simulink library "typhoonPatterns"  (R2017b)
settings: Solver=VariableStepAuto  StartTime=0.0  StopTime=10.0  RelTol=1e-3
undefined symbols (not defined in the file or in its folder): c_clamp, C_l, c_picoup_seq, crun_sp_ind, cst_sp_ind, f, f_picoup, f_sp_ind, fc, Jm, L, L1, L2, L_l, l_picoup_seq, La_DC, Ld, Lf_DC, Llr1_ind, Llr2_ind, Llr_ind, llrm_sp_ind, Lls_ind, llsa_sp_ind, llsm_sp_ind, Lm, Lq, n1, n2, nanm_sp_ind, pms, R, R1, R2, r_clamp, R_l, r_picoup_seq, Ra_DC, Rf_DC, Rm, Rr1_ind, Rr2_ind, Rr_ind, rrm_sp_ind, rrun_sp_ind, Rs, Rs_ind, rsa_sp_ind, rsm_sp_ind, rst_sp_ind
libraries: powerlib x282
(part 2 of 3)

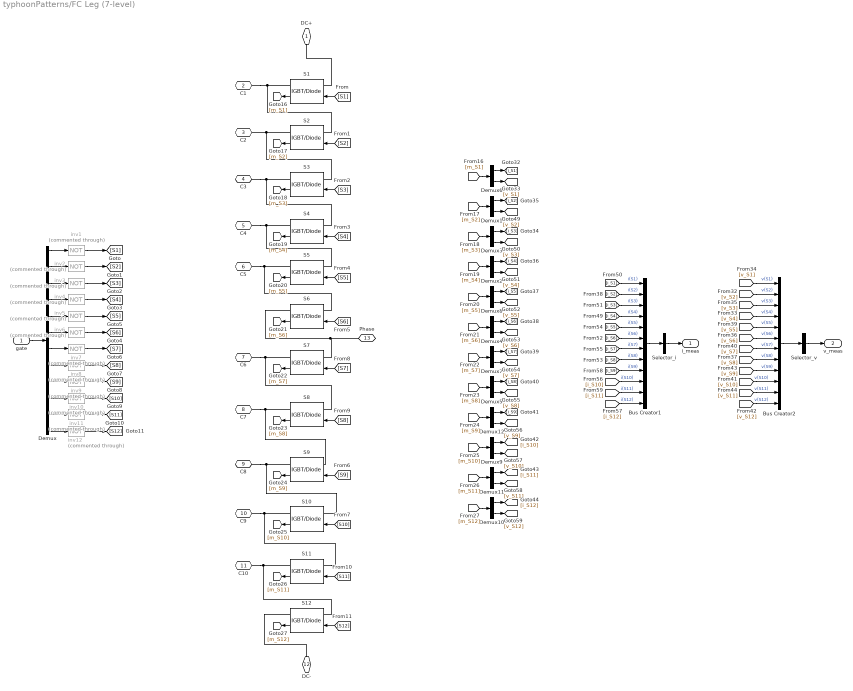
== system typhoonPatterns/FC Leg (7-level) ==
  gate : Inport
  Bus Creator1 : BusCreator  Inputs=12
  Bus Creator2 : BusCreator  Inputs=12
  Demux : Demux  Outputs=12
  Demux{1..12} (12 alike) : Demux  Outputs=2
  S{1..12} (12 alike) : powerlib/Power Electronics/IGBT//Diode  Ron=r_on  Rs=r_s  Cs=c_s  Measurements=on
  Selector_i : BusSelector  OutputSignals=i(S1)  OutputAsBus=on
  Selector_v : BusSelector  OutputSignals=v(S1)  OutputAsBus=on
  inv{1..12} (12 alike) : Logic  Commented=through  Operator=NOT  AllPortsSameDT=off  OutDataTypeStr=boolean
  DC+ : PMIOPort  Port=1  Side=Left
  C1 : PMIOPort  Port=2  Side=Left
  C2 : PMIOPort  Port=3  Side=Left
  C3 : PMIOPort  Port=4  Side=Left
  C4 : PMIOPort  Port=5  Side=Left
  C5 : PMIOPort  Port=6  Side=Left
  C6 : PMIOPort  Port=7  Side=Left
  C7 : PMIOPort  Port=8  Side=Left
  C8 : PMIOPort  Port=9  Side=Left
  C9 : PMIOPort  Port=10  Side=Left
  C10 : PMIOPort  Port=11  Side=Left
  DC- : PMIOPort  Port=12  Side=Left
  Phase : PMIOPort  Port=13  Side=Right
  i_meas : Outport
  v_meas : Outport  Port=2
  wires:
  Demux3/2 -> [v_S3]
  Demux1/1 -> [i_S2]
  [v_S7] -> Bus Creator2/7  "v(S7)"
  [v_S6] -> Bus Creator2/6  "v(S6)"
  Demux6/2 -> [v_S1]
  Demux6/1 -> [i_S1]
  [v_S1] -> Bus Creator2/1  "v(S1)"
  Bus Creator2/1 -> Selector_v/1
  Selector_v/1 -> v_meas/1
  Bus Creator1/1 -> Selector_i/1
  [v_S3] -> Bus Creator2/3  "v(S3)"
  [i_S2] -> Bus Creator1/2  "i(S2)"
  [i_S11] -> Bus Creator1/11  "i(S11)"
  [i_S4] -> Bus Creator1/4  "i(S4)"
  [i_S10] -> Bus Creator1/10  "i(S10)"
  [i_S1] -> Bus Creator1/1  "i(S1)"
  [i_S7] -> Bus Creator1/7  "i(S7)"
  [i_S5] -> Bus Creator1/5  "i(S5)"
  [i_S3] -> Bus Creator1/3  "i(S3)"
  [i_S12] -> Bus Creator1/12  "i(S12)"
  Demux7/1 -> [i_S7]
  Demux9/1 -> [i_S10]
  [m_S3] -> Demux3/1
  [v_S4] -> Bus Creator2/4  "v(S4)"
  Demux4/1 -> [i_S6]
  [m_S5] -> Demux8/1
  S2/1 -> [m_S2]
  [m_S11] -> Demux11/1
  [v_S8] -> Bus Creator2/8  "v(S8)"
  S12/1 -> [m_S12]
  S1/1 -> [m_S1]
  Demux5/1 -> [i_S8]
  Demux4/2 -> [v_S6]
  Demux2/2 -> [v_S4]
  inv7/1 -> [S7]
  inv8/1 -> [S8]
  inv6/1 -> [S6]
  inv12/1 -> [S12]
  Demux8/1 -> [i_S5]
  inv10/1 -> [S10]
  inv11/1 -> [S11]
  Demux11/1 -> [i_S11]
  Demux/1 -> inv1/1
  Demux/3 -> inv3/1
  [S5] -> S5/1
  [S6] -> S6/1
  S8/1 -> [m_S8]
  gate/1 -> Demux/1
  [S7] -> S7/1
  [i_S8] -> Bus Creator1/8  "i(S8)"
  Demux/4 -> inv4/1
  [S2] -> S2/1
  [i_S6] -> Bus Creator1/6  "i(S6)"
  Selector_i/1 -> i_meas/1
  [v_S5] -> Bus Creator2/5  "v(S5)"
  Demux/5 -> inv5/1
  [S11] -> S11/1
  [S4] -> S4/1
  Demux/12 -> inv12/1
  Demux/10 -> inv10/1
  [S9] -> S9/1
  Demux/8 -> inv8/1
  Demux/11 -> inv11/1
  Demux/9 -> inv9/1
  [i_S9] -> Bus Creator1/9  "i(S9)"
  [m_S9] -> Demux12/1
  [m_S6] -> Demux4/1
  S4/1 -> [m_S4]
  Demux1/2 -> [v_S2]
  S11/1 -> [m_S11]
  Demux/7 -> inv7/1
  [m_S8] -> Demux5/1
  Demux10/1 -> [i_S12]
  [m_S1] -> Demux6/1
  S5/1 -> [m_S5]
  [v_S10] -> Bus Creator2/10  "v(S10)"
  [v_S11] -> Bus Creator2/11  "v(S11)"
  [m_S7] -> Demux7/1
  Demux/6 -> inv6/1
  [v_S12] -> Bus Creator2/12  "v(S12)"
  S7/1 -> [m_S7]
  [m_S4] -> Demux2/1
  Demux12/2 -> [v_S9]
  inv5/1 -> [S5]
  S6/1 -> [m_S6]
  [m_S2] -> Demux1/1
  [S8] -> S8/1
  [S1] -> S1/1
  Demux3/1 -> [i_S3]
  Demux/2 -> inv2/1
  inv2/1 -> [S2]
  inv3/1 -> [S3]
  Demux5/2 -> [v_S8]
  Demux12/1 -> [i_S9]
  [v_S2] -> Bus Creator2/2  "v(S2)"
  [S10] -> S10/1
  inv1/1 -> [S1]
  S3/1 -> [m_S3]
  inv4/1 -> [S4]
  [m_S10] -> Demux9/1
  Demux10/2 -> [v_S12]
  Demux11/2 -> [v_S11]
  Demux2/1 -> [i_S4]
  [S12] -> S12/1
  Demux9/2 -> [v_S10]
  [m_S12] -> Demux10/1
  [v_S9] -> Bus Creator2/9  "v(S9)"
  Demux8/2 -> [v_S5]
  S10/1 -> [m_S10]
  Demux7/2 -> [v_S7]
  S9/1 -> [m_S9]
  [S3] -> S3/1
  inv9/1 -> [S9]
  connections:
  S7/LConn1 -- Phase/RConn1 -- S6/RConn1
  S8/LConn1 -- C6/RConn1 -- S7/RConn1
  C3/RConn1 -- S3/RConn1 -- S4/LConn1
  S8/RConn1 -- C7/RConn1 -- S9/LConn1
  C1/RConn1 -- S1/RConn1 -- S2/LConn1
  S6/LConn1 -- S5/RConn1 -- C5/RConn1
  C10/RConn1 -- S11/RConn1 -- S12/LConn1
  C2/RConn1 -- S2/RConn1 -- S3/LConn1
  S5/LConn1 -- S4/RConn1 -- C4/RConn1
  S10/LConn1 -- S9/RConn1 -- C8/RConn1
  C9/RConn1 -- S10/RConn1 -- S11/LConn1
  S1/LConn1 -- DC+/RConn1
  DC-/RConn1 -- S12/RConn1

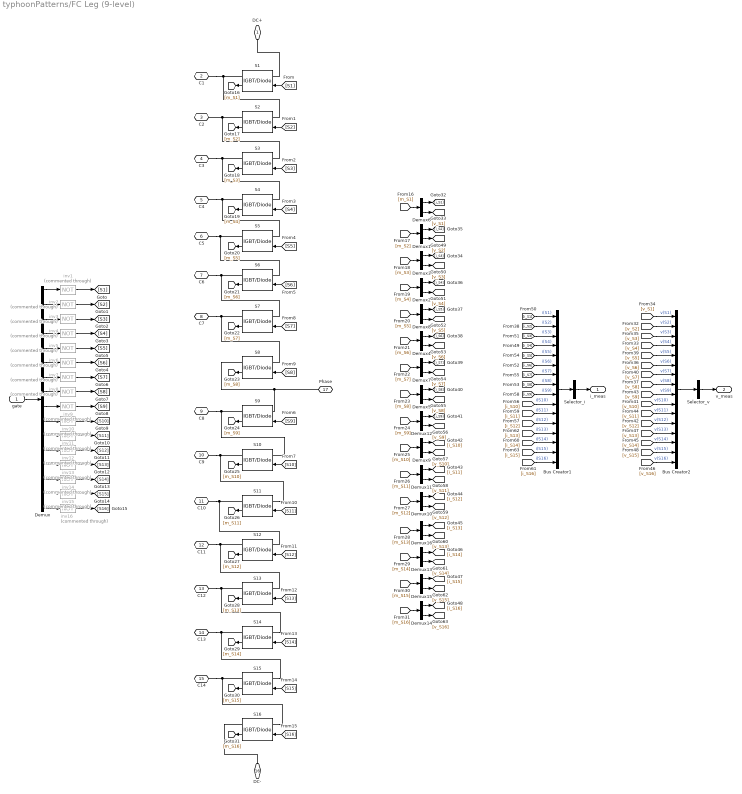
== system typhoonPatterns/FC Leg (9-level) ==
  gate : Inport
  Bus Creator1 : BusCreator  Inputs=16
  Bus Creator2 : BusCreator  Inputs=16
  Demux : Demux  Outputs=16
  Demux{1..16} (16 alike) : Demux  Outputs=2
  S{1..16} (16 alike) : powerlib/Power Electronics/IGBT//Diode  Ron=r_on  Rs=r_s  Cs=c_s  Measurements=on
  Selector_i : BusSelector  OutputSignals=i(S1)  OutputAsBus=on
  Selector_v : BusSelector  OutputSignals=v(S1)  OutputAsBus=on
  inv{1..16} (16 alike) : Logic  Commented=through  Operator=NOT  AllPortsSameDT=off  OutDataTypeStr=boolean
  DC+ : PMIOPort  Port=1  Side=Left
  C1 : PMIOPort  Port=2  Side=Left
  C2 : PMIOPort  Port=3  Side=Left
  C3 : PMIOPort  Port=4  Side=Left
  C4 : PMIOPort  Port=5  Side=Left
  C5 : PMIOPort  Port=6  Side=Left
  C6 : PMIOPort  Port=7  Side=Left
  C7 : PMIOPort  Port=8  Side=Left
  C8 : PMIOPort  Port=9  Side=Left
  C9 : PMIOPort  Port=10  Side=Left
  C10 : PMIOPort  Port=11  Side=Left
  C11 : PMIOPort  Port=12  Side=Left
  C12 : PMIOPort  Port=13  Side=Left
  C13 : PMIOPort  Port=14  Side=Left
  C14 : PMIOPort  Port=15  Side=Left
  DC- : PMIOPort  Port=16  Side=Left
  Phase : PMIOPort  Port=17  Side=Right
  i_meas : Outport
  v_meas : Outport  Port=2
  wires:
  Demux/15 -> inv15/1
  [S14] -> S14/1
  [S13] -> S13/1
  [S16] -> S16/1
  [S15] -> S15/1
  Demux/16 -> inv16/1
  Demux/14 -> inv14/1
  Demux/13 -> inv13/1
  Demux/12 -> inv12/1
  Demux/9 -> inv9/1
  Demux/2 -> inv2/1
  gate/1 -> Demux/1
  Demux/10 -> inv10/1
  [S11] -> S11/1
  [S12] -> S12/1
  Demux/8 -> inv8/1
  [S7] -> S7/1
  Demux/11 -> inv11/1
  [S8] -> S8/1
  [S5] -> S5/1
  [S3] -> S3/1
  Demux/4 -> inv4/1
  Demux/3 -> inv3/1
  [S9] -> S9/1
  Demux/7 -> inv7/1
  Demux/6 -> inv6/1
  Demux/1 -> inv1/1
  Demux/5 -> inv5/1
  [S4] -> S4/1
  [S6] -> S6/1
  [S2] -> S2/1
  [S1] -> S1/1
  [S10] -> S10/1
  inv1/1 -> [S1]
  inv3/1 -> [S3]
  inv4/1 -> [S4]
  inv2/1 -> [S2]
  inv5/1 -> [S5]
  inv8/1 -> [S8]
  inv6/1 -> [S6]
  inv7/1 -> [S7]
  inv9/1 -> [S9]
  inv11/1 -> [S11]
  inv10/1 -> [S10]
  inv12/1 -> [S12]
  inv15/1 -> [S15]
  inv13/1 -> [S13]
  inv14/1 -> [S14]
  inv16/1 -> [S16]
  S1/1 -> [m_S1]
  S2/1 -> [m_S2]
  S4/1 -> [m_S4]
  S5/1 -> [m_S5]
  S6/1 -> [m_S6]
  S3/1 -> [m_S3]
  S7/1 -> [m_S7]
  S8/1 -> [m_S8]
  S9/1 -> [m_S9]
  S10/1 -> [m_S10]
  S11/1 -> [m_S11]
  S12/1 -> [m_S12]
  S13/1 -> [m_S13]
  S14/1 -> [m_S14]
  S15/1 -> [m_S15]
  S16/1 -> [m_S16]
  [m_S1] -> Demux6/1
  Selector_v/1 -> v_meas/1
  Demux6/1 -> [i_S1]
  Bus Creator2/1 -> Selector_v/1
  [v_S1] -> Bus Creator2/1  "v(S1)"
  Selector_i/1 -> i_meas/1
  Demux6/2 -> [v_S1]
  [v_S2] -> Bus Creator2/2  "v(S2)"
  [v_S3] -> Bus Creator2/3  "v(S3)"
  [v_S4] -> Bus Creator2/4  "v(S4)"
  [v_S5] -> Bus Creator2/5  "v(S5)"
  [v_S7] -> Bus Creator2/7  "v(S7)"
  [v_S6] -> Bus Creator2/6  "v(S6)"
  [v_S8] -> Bus Creator2/8  "v(S8)"
  [v_S9] -> Bus Creator2/9  "v(S9)"
  [v_S11] -> Bus Creator2/11  "v(S11)"
  [v_S10] -> Bus Creator2/10  "v(S10)"
  [v_S12] -> Bus Creator2/12  "v(S12)"
  [v_S13] -> Bus Creator2/13  "v(S13)"
  [v_S15] -> Bus Creator2/15  "v(S15)"
  [v_S14] -> Bus Creator2/14  "v(S14)"
  [v_S16] -> Bus Creator2/16  "v(S16)"
  [i_S6] -> Bus Creator1/6  "i(S6)"
  [i_S5] -> Bus Creator1/5  "i(S5)"
  [i_S14] -> Bus Creator1/14  "i(S14)"
  [i_S7] -> Bus Creator1/7  "i(S7)"
  [i_S16] -> Bus Creator1/16  "i(S16)"
  [i_S13] -> Bus Creator1/13  "i(S13)"
  [i_S15] -> Bus Creator1/15  "i(S15)"
  [i_S1] -> Bus Creator1/1  "i(S1)"
  [i_S10] -> Bus Creator1/10  "i(S10)"
  [i_S8] -> Bus Creator1/8  "i(S8)"
  [i_S4] -> Bus Creator1/4  "i(S4)"
  [i_S11] -> Bus Creator1/11  "i(S11)"
  [i_S2] -> Bus Creator1/2  "i(S2)"
  [i_S12] -> Bus Creator1/12  "i(S12)"
  [i_S3] -> Bus Creator1/3  "i(S3)"
  [i_S9] -> Bus Creator1/9  "i(S9)"
  Bus Creator1/1 -> Selector_i/1
  Demux1/2 -> [v_S2]
  Demux1/1 -> [i_S2]
  [m_S2] -> Demux1/1
  Demux3/2 -> [v_S3]
  [m_S3] -> Demux3/1
  Demux2/1 -> [i_S4]
  Demux2/2 -> [v_S4]
  [m_S4] -> Demux2/1
  Demux8/2 -> [v_S5]
  Demux8/1 -> [i_S5]
  [m_S5] -> Demux8/1
  Demux4/1 -> [i_S6]
  Demux5/1 -> [i_S8]
  [m_S8] -> Demux5/1
  Demux4/2 -> [v_S6]
  [m_S6] -> Demux4/1
  Demux5/2 -> [v_S8]
  [m_S7] -> Demux7/1
  Demux7/2 -> [v_S7]
  Demux12/2 -> [v_S9]
  Demux12/1 -> [i_S9]
  [m_S9] -> Demux12/1
  Demux9/1 -> [i_S10]
  Demux10/1 -> [i_S12]
  [m_S12] -> Demux10/1
  Demux9/2 -> [v_S10]
  [m_S10] -> Demux9/1
  Demux10/2 -> [v_S12]
  [m_S11] -> Demux11/1
  Demux11/2 -> [v_S11]
  Demux16/2 -> [v_S13]
  Demux16/1 -> [i_S13]
  [m_S13] -> Demux16/1
  Demux13/1 -> [i_S14]
  Demux14/1 -> [i_S16]
  [m_S16] -> Demux14/1
  Demux13/2 -> [v_S14]
  [m_S14] -> Demux13/1
  Demux14/2 -> [v_S16]
  [m_S15] -> Demux15/1
  Demux15/2 -> [v_S15]
  Demux3/1 -> [i_S3]
  Demux7/1 -> [i_S7]
  Demux11/1 -> [i_S11]
  Demux15/1 -> [i_S15]
  connections:
  DC-/RConn1 -- S16/RConn1
  S1/LConn1 -- DC+/RConn1
  C1/RConn1 -- S1/RConn1 -- S2/LConn1
  S2/RConn1 -- S3/LConn1 -- C2/RConn1
  S8/RConn1 -- Phase/RConn1 -- S9/LConn1
  C3/RConn1 -- S3/RConn1 -- S4/LConn1
  S5/LConn1 -- S4/RConn1 -- C4/RConn1
  S6/LConn1 -- S5/RConn1 -- C5/RConn1
  C6/RConn1 -- S6/RConn1 -- S7/LConn1
  C7/RConn1 -- S7/RConn1 -- S8/LConn1
  S9/RConn1 -- C8/RConn1 -- S10/LConn1
  C9/RConn1 -- S10/RConn1 -- S11/LConn1
  C10/RConn1 -- S11/RConn1 -- S12/LConn1
  S13/LConn1 -- S12/RConn1 -- C11/RConn1
  S14/LConn1 -- S13/RConn1 -- C12/RConn1
  S15/LConn1 -- S14/RConn1 -- C13/RConn1
  S16/LConn1 -- S15/RConn1 -- C14/RConn1

== system typhoonPatterns/Flyback ==
  gate : Inport
  D : powerlib/Power Electronics/Diode  Ron=r_on  Lon=0  Vf=0  IC=0  UseSnubber=0  Rs=r_s  Cs=c_s  Measurements=off
  S : powerlib/Power Electronics/Mosfet  Ron=r_on  Lon=0  Rd=r_on  Vfd=0  IC=0  Rs=r_s  Cs=c_s  Measurements=off
  T : powerlib/Elements/Linear Transformer  UNITS=SI  NominalPower=[250e6 60 ]  winding1=[n1 R1 L1]  winding2=[n2 R2 L2]  ThreeWindings=off  winding3=[3.15e+05 0.7938 0.084225]  RmLm=[Rm Lm]  Measurements=None  DataType=on
  inv1 : Logic  Commented=through  Operator=NOT  AllPortsSameDT=off  OutDataTypeStr=boolean
  In+ : PMIOPort  Port=1  Side=Left
  In- : PMIOPort  Port=2  Side=Left
  Out+ : PMIOPort  Port=3  Side=Right
  Out- : PMIOPort  Port=4  Side=Right
  wires:
  inv1/1 -> S/1
  gate/1 -> inv1/1
  connections:
  In-/RConn1 -- S/RConn1
  S/LConn1 -- T/LConn2
  In+/RConn1 -- T/LConn1
  D/RConn1 -- Out+/RConn1
  D/LConn1 -- T/RConn2
  T/RConn1 -- Out-/RConn1

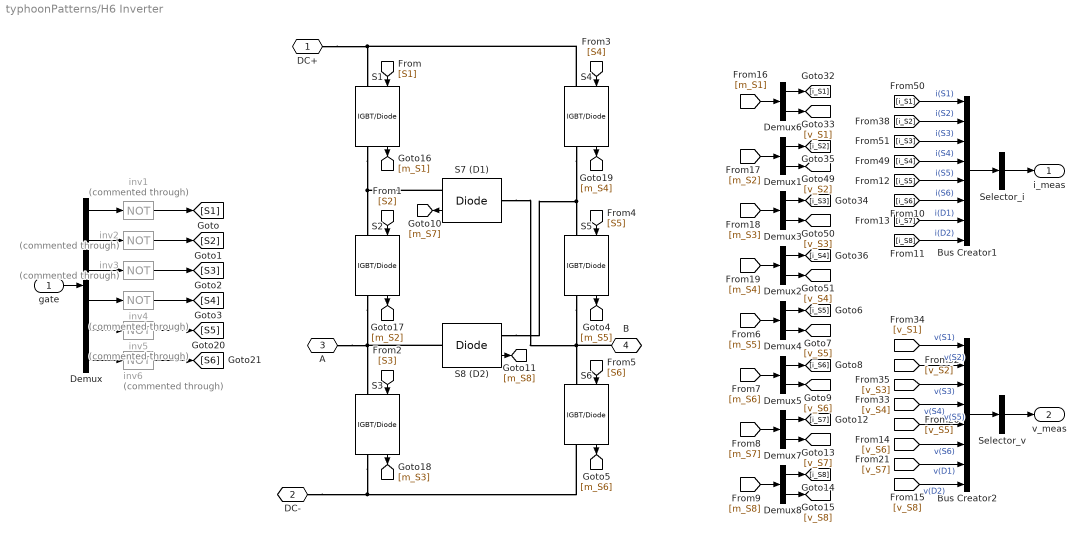
== system typhoonPatterns/H6 Inverter ==
  gate : Inport
  Bus Creator1 : BusCreator  Inputs=8
  Bus Creator2 : BusCreator  Inputs=8
  Demux : Demux  Outputs=6
  Demux{1..8} (8 alike) : Demux  Outputs=2
  S{1..6} (6 alike) : powerlib/Power Electronics/IGBT//Diode  Ron=r_on  Rs=r_s  Cs=c_s  Measurements=on
  S7 (D1) : powerlib/Power Electronics/Diode  Ron=r_on  Lon=0  Vf=v_f  IC=0  UseSnubber=0  Rs=r_s  Cs=c_s  Measurements=on
  S8 (D2) : powerlib/Power Electronics/Diode  Ron=r_on  Lon=0  Vf=v_f  IC=0  UseSnubber=0  Rs=r_s  Cs=c_s  Measurements=on
  Selector_i : BusSelector  OutputSignals=i(S1)  OutputAsBus=on
  Selector_v : BusSelector  OutputSignals=v(S1)  OutputAsBus=on
  inv{1..6} (6 alike) : Logic  Commented=through  Operator=NOT  AllPortsSameDT=off  OutDataTypeStr=boolean
  DC+ : PMIOPort  Port=1  Side=Left
  DC- : PMIOPort  Port=2  Side=Left
  A : PMIOPort  Port=3  Side=Right
  B : PMIOPort  Port=4  Side=Right
  i_meas : Outport
  v_meas : Outport  Port=2
  wires:
  Demux1/2 -> [v_S2]
  [S4] -> S4/1
  [v_S3] -> Bus Creator2/3  "v(S3)"
  [S1] -> S1/1
  Demux1/1 -> [i_S2]
  [v_S4] -> Bus Creator2/4  "v(S4)"
  gate/1 -> Demux/1
  Demux3/2 -> [v_S3]
  [v_S2] -> Bus Creator2/2  "v(S2)"
  Demux6/2 -> [v_S1]
  Demux/2 -> inv2/1
  [i_S1] -> Bus Creator1/1  "i(S1)"
  S3/1 -> [m_S3]
  inv4/1 -> [S4]
  Demux/1 -> inv1/1
  inv2/1 -> [S2]
  inv1/1 -> [S1]
  [m_S4] -> Demux2/1
  Bus Creator1/1 -> Selector_i/1
  Selector_i/1 -> i_meas/1
  Demux/3 -> inv3/1
  [m_S2] -> Demux1/1
  [S2] -> S2/1
  S2/1 -> [m_S2]
  Selector_v/1 -> v_meas/1
  [v_S1] -> Bus Creator2/1  "v(S1)"
  Demux2/2 -> [v_S4]
  [i_S4] -> Bus Creator1/4  "i(S4)"
  Demux6/1 -> [i_S1]
  [m_S1] -> Demux6/1
  [S3] -> S3/1
  [i_S2] -> Bus Creator1/2  "i(S2)"
  [i_S3] -> Bus Creator1/3  "i(S3)"
  [m_S3] -> Demux3/1
  Demux2/1 -> [i_S4]
  inv3/1 -> [S3]
  Bus Creator2/1 -> Selector_v/1
  Demux/4 -> inv4/1
  Demux3/1 -> [i_S3]
  S4/1 -> [m_S4]
  S1/1 -> [m_S1]
  [S5] -> S5/1
  S5/1 -> [m_S5]
  [S6] -> S6/1
  S6/1 -> [m_S6]
  S7 (D1)/1 -> [m_S7]
  S8 (D2)/1 -> [m_S8]
  [m_S5] -> Demux4/1
  Demux4/2 -> [v_S5]
  Demux4/1 -> [i_S5]
  [m_S6] -> Demux5/1
  Demux5/2 -> [v_S6]
  Demux5/1 -> [i_S6]
  Demux7/2 -> [v_S7]
  Demux7/1 -> [i_S7]
  [m_S7] -> Demux7/1
  Demux8/2 -> [v_S8]
  [m_S8] -> Demux8/1
  Demux8/1 -> [i_S8]
  [i_S5] -> Bus Creator1/5  "i(S5)"
  [i_S6] -> Bus Creator1/6  "i(S6)"
  [i_S7] -> Bus Creator1/7  "i(D1)"
  [i_S8] -> Bus Creator1/8  "i(D2)"
  [v_S6] -> Bus Creator2/6  "v(S6)"
  [v_S7] -> Bus Creator2/7  "v(D1)"
  [v_S5] -> Bus Creator2/5  "v(S5)"
  [v_S8] -> Bus Creator2/8  "v(D2)"
  Demux/6 -> inv6/1
  inv5/1 -> [S5]
  inv6/1 -> [S6]
  Demux/5 -> inv5/1
  connections:
  S1/RConn1 -- S2/LConn1 -- S7 (D1)/RConn1
  S2/RConn1 -- A/RConn1 -- S8 (D2)/LConn1 -- S3/LConn1
  S4/RConn1 -- S5/LConn1 -- S8 (D2)/RConn1
  S5/RConn1 -- S7 (D1)/LConn1 -- S6/LConn1 -- B/RConn1
  S3/RConn1 -- DC-/RConn1 -- S6/RConn1
  S4/LConn1 -- DC+/RConn1 -- S1/LConn1

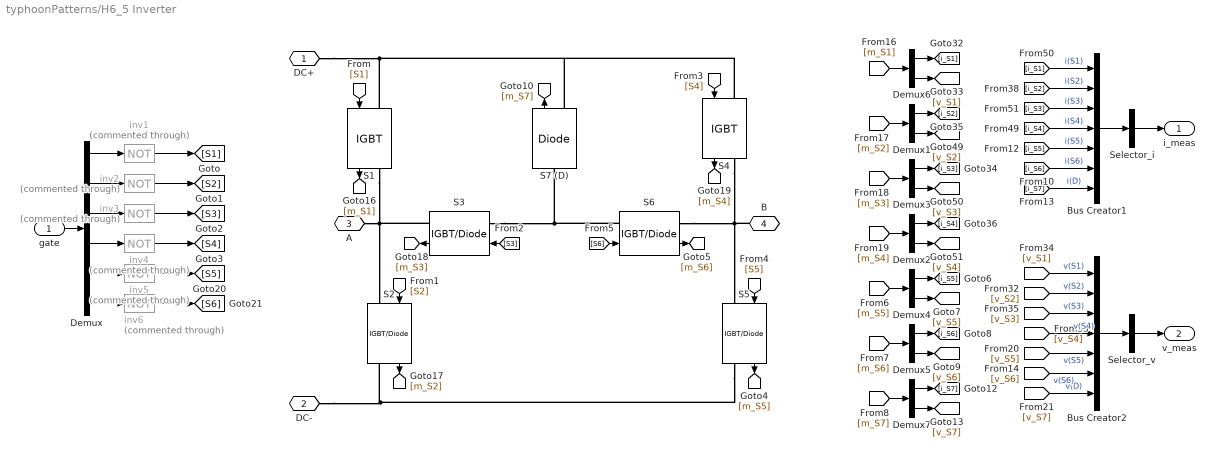
== system typhoonPatterns/H6_5 Inverter ==
  gate : Inport
  Bus Creator1 : BusCreator  Inputs=7
  Bus Creator2 : BusCreator  Inputs=7
  Demux : Demux  Outputs=6
  Demux{1..7} (7 alike) : Demux  Outputs=2
  S1 : powerlib/Power Electronics/IGBT  Ron=r_on  Lon=0  Vf=v_f  Tf=1e-6  Tt=2e-6  IC=0  Rs=r_s  Cs=c_s  Measurements=on
  S{2..3,5..6} (4 alike) : powerlib/Power Electronics/IGBT//Diode  Ron=r_on  Rs=r_s  Cs=c_s  Measurements=on
  S4 : powerlib/Power Electronics/IGBT  Ron=r_on  Lon=0  Vf=v_f  Tf=1e-6  Tt=2e-6  IC=0  Rs=r_s  Cs=c_s  Measurements=on
  S7 (D) : powerlib/Power Electronics/Diode  Ron=r_on  Lon=0  Vf=v_f  IC=0  UseSnubber=0  Rs=r_s  Cs=c_s  Measurements=on
  Selector_i : BusSelector  OutputSignals=i(S1)  OutputAsBus=on
  Selector_v : BusSelector  OutputSignals=v(S1)  OutputAsBus=on
  inv{1..6} (6 alike) : Logic  Commented=through  Operator=NOT  AllPortsSameDT=off  OutDataTypeStr=boolean
  DC+ : PMIOPort  Port=1  Side=Left
  DC- : PMIOPort  Port=2  Side=Left
  A : PMIOPort  Port=3  Side=Right
  B : PMIOPort  Port=4  Side=Right
  i_meas : Outport
  v_meas : Outport  Port=2
  wires:
  Demux/5 -> inv5/1
  inv6/1 -> [S6]
  inv5/1 -> [S5]
  Demux/6 -> inv6/1
  [v_S5] -> Bus Creator2/5  "v(S5)"
  [v_S7] -> Bus Creator2/7  "v(D)"
  [v_S6] -> Bus Creator2/6  "v(S6)"
  [i_S7] -> Bus Creator1/7  "i(D)"
  [i_S6] -> Bus Creator1/6  "i(S6)"
  [i_S5] -> Bus Creator1/5  "i(S5)"
  [m_S7] -> Demux7/1
  Demux7/1 -> [i_S7]
  Demux7/2 -> [v_S7]
  Demux5/1 -> [i_S6]
  Demux5/2 -> [v_S6]
  [m_S6] -> Demux5/1
  Demux4/1 -> [i_S5]
  Demux4/2 -> [v_S5]
  [m_S5] -> Demux4/1
  S7 (D)/1 -> [m_S7]
  S5/1 -> [m_S5]
  [S5] -> S5/1
  S1/1 -> [m_S1]
  S4/1 -> [m_S4]
  Demux3/1 -> [i_S3]
  Demux/4 -> inv4/1
  Bus Creator2/1 -> Selector_v/1
  inv3/1 -> [S3]
  Demux2/1 -> [i_S4]
  [m_S3] -> Demux3/1
  [i_S3] -> Bus Creator1/3  "i(S3)"
  [i_S2] -> Bus Creator1/2  "i(S2)"
  [S3] -> S3/1
  [m_S1] -> Demux6/1
  Demux6/1 -> [i_S1]
  [i_S4] -> Bus Creator1/4  "i(S4)"
  Demux2/2 -> [v_S4]
  [v_S1] -> Bus Creator2/1  "v(S1)"
  Selector_v/1 -> v_meas/1
  S2/1 -> [m_S2]
  [S2] -> S2/1
  [m_S2] -> Demux1/1
  Demux/3 -> inv3/1
  Selector_i/1 -> i_meas/1
  Bus Creator1/1 -> Selector_i/1
  [m_S4] -> Demux2/1
  inv1/1 -> [S1]
  inv2/1 -> [S2]
  Demux/1 -> inv1/1
  inv4/1 -> [S4]
  S3/1 -> [m_S3]
  [i_S1] -> Bus Creator1/1  "i(S1)"
  Demux/2 -> inv2/1
  Demux6/2 -> [v_S1]
  [v_S2] -> Bus Creator2/2  "v(S2)"
  Demux3/2 -> [v_S3]
  gate/1 -> Demux/1
  [v_S4] -> Bus Creator2/4  "v(S4)"
  Demux1/1 -> [i_S2]
  [S1] -> S1/1
  [v_S3] -> Bus Creator2/3  "v(S3)"
  [S4] -> S4/1
  Demux1/2 -> [v_S2]
  S6/1 -> [m_S6]
  [S6] -> S6/1
  connections:
  DC+/RConn1 -- S4/LConn1 -- S7 (D)/RConn1 -- S1/LConn1
  S4/RConn1 -- S6/RConn1 -- B/RConn1 -- S5/LConn1
  S5/RConn1 -- DC-/RConn1 -- S2/RConn1
  S1/RConn1 -- A/RConn1 -- S3/RConn1 -- S2/LConn1
  S3/LConn1 -- S6/LConn1 -- S7 (D)/LConn1

== system typhoonPatterns/IGBT Leg ==
  gates : Inport
  Bus Creator : BusCreator  Inputs=2
  Bus Creator1 : BusCreator  Inputs=2
  Demux1 : Demux  Outputs=2
  Demux2 : Demux  Outputs=2
  Demux4 : Demux  Outputs=2
  S1 : powerlib/Power Electronics/IGBT//Diode  Ron=r_on  Rs=r_s  Cs=c_s  Measurements=on
  S2 : powerlib/Power Electronics/IGBT//Diode  Ron=r_on  Rs=r_s  Cs=c_s  Measurements=on
  Selector_i : BusSelector  OutputSignals=i(S1)  OutputAsBus=on
  Selector_v : BusSelector  OutputSignals=v(S1)  OutputAsBus=on
  inv1 : Logic  Commented=through  Operator=NOT  AllPortsSameDT=off  OutDataTypeStr=boolean
  inv2 : Logic  Commented=through  Operator=NOT  AllPortsSameDT=off  OutDataTypeStr=boolean
  DC+ : PMIOPort  Port=1  Side=Left
  DC- : PMIOPort  Port=2  Side=Left
  Phase : PMIOPort  Port=3  Side=Right
  i_meas : Outport
  v_meas : Outport  Port=2
  wires:
  Demux1/1 -> [i_S1]
  Demux2/1 -> [i_S2]
  Demux2/2 -> [v_S2]
  [m_S2] -> Demux2/1
  Selector_i/1 -> i_meas/1
  Bus Creator/1 -> Selector_i/1
  [m_S1] -> Demux1/1
  Demux1/2 -> [v_S1]
  [i_S1] -> Bus Creator/1  "i(S1)"
  [v_S1] -> Bus Creator1/1  "v(S1)"
  Selector_v/1 -> v_meas/1
  [v_S2] -> Bus Creator1/2  "v(S2)"
  [i_S2] -> Bus Creator/2  "i(S2)"
  Bus Creator1/1 -> Selector_v/1
  inv2/1 -> [S2]
  gates/1 -> Demux4/1
  Demux4/1 -> inv1/1
  inv1/1 -> [S1]
  Demux4/2 -> inv2/1
  [S1] -> S1/1
  [S2] -> S2/1
  S1/1 -> [m_S1]
  S2/1 -> [m_S2]
  connections:
  S2/RConn1 -- DC-/RConn1
  S2/LConn1 -- Phase/RConn1 -- S1/RConn1
  S1/LConn1 -- DC+/RConn1

== system typhoonPatterns/Ideal Transformer ==
  T1 : powerlib/Elements/Linear Transformer  UNITS=SI  NominalPower=[1, 60]  winding1=[n1, 0, 0]  winding2=[n2, 0, 0]  ThreeWindings=off  winding3=[ 315e3 0.002 0.08 ]  RmLm=[0.001, inf]  Measurements=None  DataType=off
      settings: AttributesFormatString=%<MaskType>
  prm_1 : PMIOPort  Port=1  Side=Left
  prm_2 : PMIOPort  Port=2  Side=Left
  sec_1 : PMIOPort  Port=3  Side=Right
  sec_2 : PMIOPort  Port=4  Side=Right
  connections:
  T1/LConn1 -- prm_1/RConn1
  T1/RConn1 -- sec_1/RConn1
  T1/LConn2 -- prm_2/RConn1
  T1/RConn2 -- sec_2/RConn1

== system typhoonPatterns/Induction Machine ==
  mech : Inport
  Asynchronous Machine1 : powerlib/Machines/Asynchronous Machine SI Units  RotorType=Squirrel-cage  PresetModel=No  MechanicalLoad=Torque Tm  ShowDetailedParameters=on  ReferenceFrame=Rotor  Units=SI  MeasurementBus=off  NominalParameters=[1 1 50]  Stator=[Rs_ind Lls_ind]  Rotor=[Rr_ind Llr_ind]  Cage1=[Rr1_ind Llr1_ind]  Cage2=[Rr2_ind Llr2_ind]  Lm=Lm_ind  Mechanical=[Jm fc pms]  PolePairs=2  InitialConditions=[0 0 0 0 0 0 0 0]  SimulateSaturation=off  Saturation=[14.03593122, 27.81365428, 53.79336849, 72.68890987, 97.98006896, 148.6815601, 215.7428561, 302.9841135, 428.7778367 ; 230, 322, 414, 460, 506, 552, 598, 644, 690]  LoadFlowParameters=1492000  TsPowergui=0  TsBlock=-1  IterativeModel=Trapezoidal non iterative  IterativeDiscreteModel=Trapezoidal non iterative  Pmec=0
  A : PMIOPort  Port=1  Side=Left
  B : PMIOPort  Port=2  Side=Left
  C : PMIOPort  Port=3  Side=Left
  meas : Outport
  wires:
  Asynchronous Machine1/1 -> meas/1
  mech/1 -> Asynchronous Machine1/1
  connections:
  Asynchronous Machine1/LConn3 -- C/RConn1
  Asynchronous Machine1/LConn2 -- B/RConn1
  Asynchronous Machine1/LConn1 -- A/RConn1

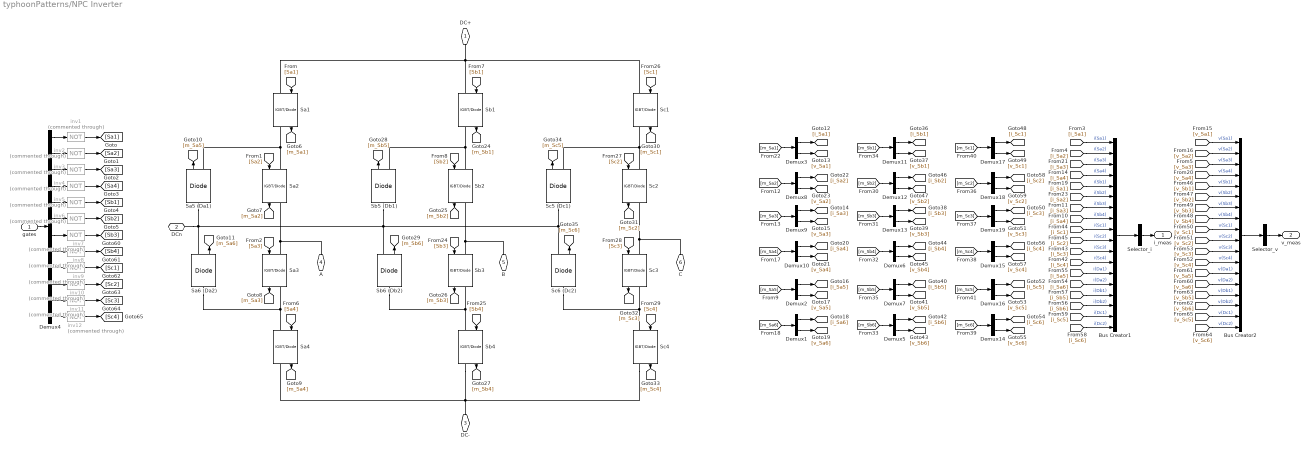
== system typhoonPatterns/NPC Inverter ==
  gates : Inport
  Bus Creator1 : BusCreator  Inputs=18
  Bus Creator2 : BusCreator  Inputs=18
  Demux{1..3,5..19} (18 alike) : Demux  Outputs=2
  Demux4 : Demux  Outputs=12
  Sa{1..4} (4 alike) : powerlib/Power Electronics/IGBT//Diode  Ron=r_on  Rs=r_s  Cs=c_s  Measurements=on
  Sa5 (Da1) : powerlib/Power Electronics/Diode  Ron=r_on  Lon=0  Vf=v_f  IC=0  UseSnubber=0  Rs=r_s  Cs=c_s  Measurements=on
  Sa6 (Da2) : powerlib/Power Electronics/Diode  Ron=r_on  Lon=0  Vf=v_f  IC=0  UseSnubber=0  Rs=r_s  Cs=c_s  Measurements=on
  Sb{1..4} (4 alike) : powerlib/Power Electronics/IGBT//Diode  Ron=r_on  Rs=r_s  Cs=c_s  Measurements=on
  Sb5 (Db1) : powerlib/Power Electronics/Diode  Ron=r_on  Lon=0  Vf=v_f  IC=0  UseSnubber=0  Rs=r_s  Cs=c_s  Measurements=on
  Sb6 (Db2) : powerlib/Power Electronics/Diode  Ron=r_on  Lon=0  Vf=v_f  IC=0  UseSnubber=0  Rs=r_s  Cs=c_s  Measurements=on
  Sc{1..4} (4 alike) : powerlib/Power Electronics/IGBT//Diode  Ron=r_on  Rs=r_s  Cs=c_s  Measurements=on
  Sc5 (Dc1) : powerlib/Power Electronics/Diode  Ron=r_on  Lon=0  Vf=v_f  IC=0  UseSnubber=0  Rs=r_s  Cs=c_s  Measurements=on
  Sc6 (Dc2) : powerlib/Power Electronics/Diode  Ron=r_on  Lon=0  Vf=v_f  IC=0  UseSnubber=0  Rs=r_s  Cs=c_s  Measurements=on
  Selector_i : BusSelector  OutputSignals=i(Sa1)  OutputAsBus=on
  Selector_v : BusSelector  OutputSignals=v(Sa1)  OutputAsBus=on
  inv{1..12} (12 alike) : Logic  Commented=through  Operator=NOT  AllPortsSameDT=off  OutDataTypeStr=boolean
  DC+ : PMIOPort  Port=1  Side=Left
  DCn : PMIOPort  Port=2  Side=Left
  DC- : PMIOPort  Port=3  Side=Left
  A : PMIOPort  Port=4  Side=Right
  B : PMIOPort  Port=5  Side=Right
  C : PMIOPort  Port=6  Side=Right
  i_meas : Outport
  v_meas : Outport  Port=2
  wires:
  [i_Sa2] -> Bus Creator1/2  "i(Sa2)"
  [m_Sa1] -> Demux3/1
  Demux4/2 -> inv2/1
  Selector_i/1 -> i_meas/1
  [m_Sa6] -> Demux1/1
  [v_Sa2] -> Bus Creator2/2  "v(Sa2)"
  Bus Creator1/1 -> Selector_i/1
  Demux2/2 -> [v_Sa5]
  [m_Sa5] -> Demux2/1
  Demux10/1 -> [i_Sa4]
  [m_Sa4] -> Demux10/1
  [m_Sa3] -> Demux9/1
  Demux2/1 -> [i_Sa5]
  [m_Sa2] -> Demux8/1
  Demux4/4 -> inv4/1
  Demux10/2 -> [v_Sa4]
  Demux4/5 -> inv5/1
  [i_Sa3] -> Bus Creator1/3  "i(Sa3)"
  Demux8/2 -> [v_Sa2]
  [v_Sa1] -> Bus Creator2/1  "v(Sa1)"
  Demux9/1 -> [i_Sa3]
  Demux9/2 -> [v_Sa3]
  [i_Sa1] -> Bus Creator1/1  "i(Sa1)"
  Bus Creator2/1 -> Selector_v/1
  Demux8/1 -> [i_Sa2]
  Demux4/6 -> inv6/1
  Demux4/1 -> inv1/1
  inv6/1 -> [Sb2]
  gates/1 -> Demux4/1
  inv3/1 -> [Sa3]
  inv5/1 -> [Sb1]
  inv1/1 -> [Sa1]
  Demux1/2 -> [v_Sa6]
  inv2/1 -> [Sa2]
  Demux3/2 -> [v_Sa1]
  [i_Sa4] -> Bus Creator1/4  "i(Sa4)"
  inv4/1 -> [Sa4]
  [v_Sa3] -> Bus Creator2/3  "v(Sa3)"
  [v_Sa4] -> Bus Creator2/4  "v(Sa4)"
  Demux4/3 -> inv3/1
  Demux3/1 -> [i_Sa1]
  Demux1/1 -> [i_Sa6]
  Selector_v/1 -> v_meas/1
  [Sa4] -> Sa4/1
  [Sa3] -> Sa3/1
  Sa5 (Da1)/1 -> [m_Sa5]
  Sa3/1 -> [m_Sa3]
  [Sa1] -> Sa1/1
  Sa2/1 -> [m_Sa2]
  Sa4/1 -> [m_Sa4]
  Sa1/1 -> [m_Sa1]
  [Sa2] -> Sa2/1
  Sa6 (Da2)/1 -> [m_Sa6]
  [Sb4] -> Sb4/1
  [Sb3] -> Sb3/1
  Sb5 (Db1)/1 -> [m_Sb5]
  Sb3/1 -> [m_Sb3]
  [Sb1] -> Sb1/1
  Sb2/1 -> [m_Sb2]
  Sb4/1 -> [m_Sb4]
  Sb1/1 -> [m_Sb1]
  [Sb2] -> Sb2/1
  Sb6 (Db2)/1 -> [m_Sb6]
  [Sc4] -> Sc4/1
  [Sc3] -> Sc3/1
  Sc5 (Dc1)/1 -> [m_Sc5]
  Sc3/1 -> [m_Sc3]
  [Sc1] -> Sc1/1
  Sc2/1 -> [m_Sc2]
  Sc4/1 -> [m_Sc4]
  Sc1/1 -> [m_Sc1]
  [Sc2] -> Sc2/1
  Sc6 (Dc2)/1 -> [m_Sc6]
  [m_Sb3] -> Demux13/1
  Demux5/1 -> [i_Sb6]
  [m_Sb5] -> Demux7/1
  Demux12/1 -> [i_Sb2]
  Demux5/2 -> [v_Sb6]
  Demux6/2 -> [v_Sb4]
  [m_Sb4] -> Demux6/1
  Demux12/2 -> [v_Sb2]
  Demux11/2 -> [v_Sb1]
  Demux7/1 -> [i_Sb5]
  Demux13/2 -> [v_Sb3]
  Demux7/2 -> [v_Sb5]
  [m_Sb6] -> Demux5/1
  Demux13/1 -> [i_Sb3]
  [m_Sb1] -> Demux11/1
  [m_Sb2] -> Demux12/1
  Demux6/1 -> [i_Sb4]
  Demux11/1 -> [i_Sb1]
  [m_Sc3] -> Demux19/1
  Demux14/1 -> [i_Sc6]
  [m_Sc5] -> Demux16/1
  Demux18/1 -> [i_Sc2]
  Demux14/2 -> [v_Sc6]
  Demux15/2 -> [v_Sc4]
  [m_Sc4] -> Demux15/1
  Demux18/2 -> [v_Sc2]
  Demux17/2 -> [v_Sc1]
  Demux16/1 -> [i_Sc5]
  Demux19/2 -> [v_Sc3]
  Demux16/2 -> [v_Sc5]
  [m_Sc6] -> Demux14/1
  Demux19/1 -> [i_Sc3]
  [m_Sc1] -> Demux17/1
  [m_Sc2] -> Demux18/1
  Demux15/1 -> [i_Sc4]
  Demux17/1 -> [i_Sc1]
  Demux4/12 -> inv12/1
  inv8/1 -> [Sb4]
  Demux4/10 -> inv10/1
  inv11/1 -> [Sc3]
  inv12/1 -> [Sc4]
  inv10/1 -> [Sc2]
  inv7/1 -> [Sb3]
  Demux4/8 -> inv8/1
  Demux4/9 -> inv9/1
  Demux4/11 -> inv11/1
  Demux4/7 -> inv7/1
  inv9/1 -> [Sc1]
  [i_Sa5] -> Bus Creator1/13  "i(Da1)"
  [i_Sa6] -> Bus Creator1/14  "i(Da2)"
  [i_Sb5] -> Bus Creator1/15  "i(Db1)"
  [i_Sb6] -> Bus Creator1/16  "i(Db2)"
  [i_Sc6] -> Bus Creator1/18  "i(Dc2)"
  [i_Sc5] -> Bus Creator1/17  "i(Dc1)"
  [i_Sa1] -> Bus Creator1/5  "i(Sb1)"
  [i_Sa2] -> Bus Creator1/6  "i(Sb2)"
  [i_Sa3] -> Bus Creator1/7  "i(Sb3)"
  [i_Sa4] -> Bus Creator1/8  "i(Sb4)"
  [i_Sc4] -> Bus Creator1/12  "i(Sc4)"
  [i_Sc1] -> Bus Creator1/9  "i(Sc1)"
  [i_Sc2] -> Bus Creator1/10  "i(Sc2)"
  [i_Sc3] -> Bus Creator1/11  "i(Sc3)"
  [v_Sa5] -> Bus Creator2/13  "v(Da1)"
  [v_Sa6] -> Bus Creator2/14  "v(Da2)"
  [v_Sb6] -> Bus Creator2/16  "v(Db2)"
  [v_Sb5] -> Bus Creator2/15  "v(Db1)"
  [v_Sc5] -> Bus Creator2/17  "v(Dc1)"
  [v_Sc6] -> Bus Creator2/18  "v(Dc2)"
  [v_Sb4] -> Bus Creator2/8  "v(Sb4)"
  [v_Sb2] -> Bus Creator2/6  "v(Sb2)"
  [v_Sb1] -> Bus Creator2/5  "v(Sb1)"
  [v_Sb3] -> Bus Creator2/7  "v(Sb3)"
  [v_Sc2] -> Bus Creator2/10  "v(Sc2)"
  [v_Sc4] -> Bus Creator2/12  "v(Sc4)"
  [v_Sc3] -> Bus Creator2/11  "v(Sc3)"
  [v_Sc1] -> Bus Creator2/9  "v(Sc1)"
  connections:
  A/RConn1 -- Sa2/RConn1 -- Sa3/LConn1
  Sa3/RConn1 -- Sa4/LConn1 -- Sa6 (Da2)/LConn1
  Sa1/RConn1 -- Sa2/LConn1 -- Sa5 (Da1)/RConn1
  Sa1/LConn1 -- Sc1/LConn1 -- Sb1/LConn1 -- DC+/RConn1
  DC-/RConn1 -- Sa4/RConn1 -- Sb4/RConn1 -- Sc4/RConn1
  B/RConn1 -- Sb2/RConn1 -- Sb3/LConn1
  Sb3/RConn1 -- Sb4/LConn1 -- Sb6 (Db2)/LConn1
  Sb1/RConn1 -- Sb2/LConn1 -- Sb5 (Db1)/RConn1
  Sc6 (Dc2)/RConn1 -- DCn/RConn1 -- Sa5 (Da1)/LConn1 -- Sa6 (Da2)/RConn1 -- Sb6 (Db2)/RConn1 -- Sb5 (Db1)/LConn1 -- Sc5 (Dc1)/LConn1
  C/RConn1 -- Sc3/LConn1 -- Sc2/RConn1
  Sc3/RConn1 -- Sc4/LConn1 -- Sc6 (Dc2)/LConn1
  Sc1/RConn1 -- Sc2/LConn1 -- Sc5 (Dc1)/RConn1

== system typhoonPatterns/NPC Leg ==
  gate : Inport
  Bus Creator : BusCreator  Inputs=6
  Bus Creator1 : BusCreator  Inputs=6
  Demux1 : Demux
  Demux{2..7} (6 alike) : Demux  Outputs=2
  S{1..4} (4 alike) : powerlib/Power Electronics/IGBT//Diode  Ron=r_on  Rs=r_s  Cs=c_s  Measurements=on
  S5 (D1) : powerlib/Power Electronics/Diode  Ron=r_on  Lon=0  Vf=v_f  IC=0  UseSnubber=0  Rs=r_s  Cs=c_s  Measurements=on
  S6 (D2) : powerlib/Power Electronics/Diode  Ron=r_on  Lon=0  Vf=v_f  IC=0  UseSnubber=0  Rs=r_s  Cs=c_s  Measurements=on
  Selector_i : BusSelector  OutputSignals=i(S1)  OutputAsBus=on
  Selector_v : BusSelector  OutputSignals=v(S1)  OutputAsBus=on
  inv{1..4} (4 alike) : Logic  Commented=through  Operator=NOT  AllPortsSameDT=off  OutDataTypeStr=boolean
  DC+ : PMIOPort  Port=1  Side=Left
  DCn : PMIOPort  Port=2  Side=Left
  DC- : PMIOPort  Port=3  Side=Left
  Phase : PMIOPort  Port=4  Side=Right
  i_meas : Outport
  v_meas : Outport  Port=2
  wires:
  [S3] -> S3/1
  [S4] -> S4/1
  [S2] -> S2/1
  [S1] -> S1/1
  Demux1/2 -> inv2/1
  gate/1 -> Demux1/1
  inv3/1 -> [S3]
  Demux1/1 -> inv1/1
  inv4/1 -> [S4]
  inv1/1 -> [S1]
  Demux1/4 -> inv4/1
  inv2/1 -> [S2]
  Demux1/3 -> inv3/1
  [v_S4] -> Bus Creator1/4  "v(S4)"
  Demux2/1 -> [i_S1]
  [m_S2] -> Demux3/1
  Demux3/1 -> [i_S2]
  Selector_i/1 -> i_meas/1
  [i_S1] -> Bus Creator/1  "i(S1)"
  Selector_v/1 -> v_meas/1
  Demux2/2 -> [v_S1]
  [m_S1] -> Demux2/1
  Demux3/2 -> [v_S2]
  Bus Creator1/1 -> Selector_v/1
  [i_S2] -> Bus Creator/2  "i(S2)"
  [v_S1] -> Bus Creator1/1  "v(S1)"
  [v_S2] -> Bus Creator1/2  "v(S2)"
  [i_S3] -> Bus Creator/3  "i(S3)"
  [m_S4] -> Demux5/1
  [i_S4] -> Bus Creator/4  "i(S4)"
  [m_S3] -> Demux4/1
  Demux5/1 -> [i_S4]
  Demux5/2 -> [v_S4]
  Bus Creator/1 -> Selector_i/1
  Demux4/2 -> [v_S3]
  [v_S3] -> Bus Creator1/3  "v(S3)"
  Demux4/1 -> [i_S3]
  S1/1 -> [m_S1]
  S2/1 -> [m_S2]
  S3/1 -> [m_S3]
  S4/1 -> [m_S4]
  [m_S6] -> Demux7/1
  Demux6/2 -> [v_S5]
  Demux7/2 -> [v_S6]
  Demux6/1 -> [i_S5]
  Demux7/1 -> [i_S6]
  [m_S5] -> Demux6/1
  [i_S6] -> Bus Creator/6  "i(D2)"
  [i_S5] -> Bus Creator/5  "i(D1)"
  [v_S6] -> Bus Creator1/6  "v(D2)"
  [v_S5] -> Bus Creator1/5  "v(D1)"
  S5 (D1)/1 -> [m_S5]
  S6 (D2)/1 -> [m_S6]
  connections:
  DC-/RConn1 -- S4/RConn1
  DCn/RConn1 -- S5 (D1)/LConn1 -- S6 (D2)/RConn1
  S4/LConn1 -- S6 (D2)/LConn1 -- S3/RConn1
  S3/LConn1 -- Phase/RConn1 -- S2/RConn1
  S2/LConn1 -- S5 (D1)/RConn1 -- S1/RConn1
  S1/LConn1 -- DC+/RConn1

== system typhoonPatterns/NPC T-type Leg ==
  gate : Inport
  Bus Creator : BusCreator  Inputs=4
  Bus Creator1 : BusCreator  Inputs=4
  Demux : Demux
  Demux{1..4} (4 alike) : Demux  Outputs=2
  S{1..4} (4 alike) : powerlib/Power Electronics/IGBT//Diode  Ron=r_on  Rs=r_s  Cs=c_s  Measurements=on
  Selector_i : BusSelector  OutputSignals=i(S1)  OutputAsBus=on
  Selector_v : BusSelector  OutputSignals=v(S1)  OutputAsBus=on
  inv{1..4} (4 alike) : Logic  Commented=through  Operator=NOT  AllPortsSameDT=off  OutDataTypeStr=boolean
  DC+ : PMIOPort  Port=1  Side=Left
  DCn : PMIOPort  Port=2  Side=Left
  DC- : PMIOPort  Port=3  Side=Left
  Phase : PMIOPort  Port=4  Side=Right
  i_meas : Outport
  v_meas : Outport  Port=2
  wires:
  [S3] -> S3/1
  [S2] -> S2/1
  [S4] -> S4/1
  [S1] -> S1/1
  Demux/4 -> inv4/1
  Demux/3 -> inv3/1
  Demux/2 -> inv2/1
  Demux/1 -> inv1/1
  gate/1 -> Demux/1
  Bus Creator1/1 -> Selector_v/1
  [v_S1] -> Bus Creator1/1  "v(S1)"
  [i_S2] -> Bus Creator/2  "i(S2)"
  [v_S2] -> Bus Creator1/2  "v(S2)"
  Bus Creator/1 -> Selector_i/1
  [m_S1] -> Demux1/1
  [i_S1] -> Bus Creator/1  "i(S1)"
  Selector_v/1 -> v_meas/1
  [m_S2] -> Demux2/1
  Demux1/2 -> [v_S1]
  Selector_i/1 -> i_meas/1
  Demux2/2 -> [v_S2]
  Demux2/1 -> [i_S2]
  Demux1/1 -> [i_S1]
  inv1/1 -> [S1]
  inv2/1 -> [S2]
  inv3/1 -> [S3]
  inv4/1 -> [S4]
  Demux3/1 -> [i_S3]
  [m_S4] -> Demux4/1
  Demux4/1 -> [i_S4]
  Demux3/2 -> [v_S3]
  [m_S3] -> Demux3/1
  Demux4/2 -> [v_S4]
  S2/1 -> [m_S2]
  S3/1 -> [m_S3]
  S1/1 -> [m_S1]
  S4/1 -> [m_S4]
  [i_S3] -> Bus Creator/3  "i(S3)"
  [i_S4] -> Bus Creator/4  "i(S4)"
  [v_S4] -> Bus Creator1/4  "v(S4)"
  [v_S3] -> Bus Creator1/3  "v(S3)"
  connections:
  DCn/RConn1 -- S2/LConn1
  S1/RConn1 -- S4/LConn1 -- Phase/RConn1 -- S3/LConn1
  S2/RConn1 -- S3/RConn1
  S4/RConn1 -- DC-/RConn1
  S1/LConn1 -- DC+/RConn1

== system typhoonPatterns/PI 2PH ==
  Pi1 : powerlib/Elements/Pi Section Line  LConnTagsString=__new0  RConnTagsString=__new0  Frequency=f  Resistance=R_l  Inductance=L_l  Capacitance=C_l  Length=length  PiSections=num_pi  Measurements=None
      settings: AttributesFormatString=\n  SourceProductName=Simscape Power Systems  SourceProductBaseCode=PS
  Pi2 : powerlib/Elements/Pi Section Line  LConnTagsString=__new0  RConnTagsString=__new0  Frequency=f  Resistance=R_l  Inductance=L_l  Capacitance=C_l  Length=length  PiSections=num_pi  Measurements=None
      settings: AttributesFormatString=\n  SourceProductName=Simscape Power Systems  SourceProductBaseCode=PS
  a_in : PMIOPort  Port=1  Side=Left
  a_out : PMIOPort  Port=2  Side=Right
  b_in : PMIOPort  Port=3  Side=Left
  b_out : PMIOPort  Port=4  Side=Right
  connections:
  Pi2/RConn1 -- b_out/RConn1
  Pi1/RConn1 -- a_out/RConn1
  Pi1/LConn1 -- a_in/RConn1
  Pi2/LConn1 -- b_in/RConn1

== system typhoonPatterns/PI 3PH ==
  Pi1 : powerlib/Elements/Pi Section Line  LConnTagsString=__new0  RConnTagsString=__new0  Frequency=f  Resistance=R_l  Inductance=L_l  Capacitance=C_l  Length=length  PiSections=num_pi  Measurements=None
      settings: AttributesFormatString=\n  SourceProductName=Simscape Power Systems  SourceProductBaseCode=PS
  Pi2 : powerlib/Elements/Pi Section Line  LConnTagsString=__new0  RConnTagsString=__new0  Frequency=f  Resistance=R_l  Inductance=L_l  Capacitance=C_l  Length=length  PiSections=num_pi  Measurements=None
      settings: AttributesFormatString=\n  SourceProductName=Simscape Power Systems  SourceProductBaseCode=PS
  Pi3 : powerlib/Elements/Pi Section Line  LConnTagsString=__new0  RConnTagsString=__new0  Frequency=f  Resistance=R_l  Inductance=L_l  Capacitance=C_l  Length=length  PiSections=num_pi  Measurements=None
      settings: AttributesFormatString=\n  SourceProductName=Simscape Power Systems  SourceProductBaseCode=PS
  a_in : PMIOPort  Port=1  Side=Left
  a_out : PMIOPort  Port=2  Side=Right
  b_in : PMIOPort  Port=3  Side=Left
  b_out : PMIOPort  Port=4  Side=Right
  c_in : PMIOPort  Port=5  Side=Left
  c_out : PMIOPort  Port=6  Side=Right
  connections:
  Pi3/RConn1 -- c_out/RConn1
  Pi3/LConn1 -- c_in/RConn1
  Pi2/LConn1 -- b_in/RConn1
  Pi1/LConn1 -- a_in/RConn1
  Pi1/RConn1 -- a_out/RConn1
  Pi2/RConn1 -- b_out/RConn1

== system typhoonPatterns/PI 3PH Seq ==
  Three-Phase PI Section Line : powerlib/Elements/Three-Phase PI Section Line  LConnTagsString=a|b|c  RConnTagsString=A|B|C  Frequency=f_picoup  Resistances=[r_picoup_seq(2) r_picoup_seq(1)]  Inductances=[l_picoup_seq(2) l_picoup_seq(1)]  Capacitances=[c_picoup_seq(2) c_picoup_seq(1)]  Length=length_picoup
      settings: SourceProductName=Simscape Power Systems
  a_in : PMIOPort  Port=1  Side=Left
  a_out : PMIOPort  Port=2  Side=Right
  b_in : PMIOPort  Port=3  Side=Left
  b_out : PMIOPort  Port=4  Side=Right
  c_in : PMIOPort  Port=5  Side=Left
  c_out : PMIOPort  Port=6  Side=Right
  connections:
  Three-Phase PI Section Line/RConn2 -- b_out/RConn1
  Three-Phase PI Section Line/RConn1 -- a_out/RConn1
  Three-Phase PI Section Line/LConn1 -- a_in/RConn1
  Three-Phase PI Section Line/LConn2 -- b_in/RConn1
  Three-Phase PI Section Line/LConn3 -- c_in/RConn1
  Three-Phase PI Section Line/RConn3 -- c_out/RConn1

== system typhoonPatterns/PI 4PH ==
  Pi{1..4} (4 alike) : powerlib/Elements/Pi Section Line  LConnTagsString=__new0  RConnTagsString=__new0  Frequency=f  Resistance=R_l  Inductance=L_l  Capacitance=C_l  Length=length  PiSections=num_pi  Measurements=None
      settings: AttributesFormatString=\n  SourceProductName=Simscape Power Systems  SourceProductBaseCode=PS
  a_in : PMIOPort  Port=1  Side=Left
  a_out : PMIOPort  Port=2  Side=Right
  b_in : PMIOPort  Port=3  Side=Left
  b_out : PMIOPort  Port=4  Side=Right
  c_in : PMIOPort  Port=5  Side=Left
  c_out : PMIOPort  Port=6  Side=Right
  d_in : PMIOPort  Port=7  Side=Left
  d_out : PMIOPort  Port=8  Side=Right
  connections:
  Pi2/RConn1 -- b_out/RConn1
  Pi1/RConn1 -- a_out/RConn1
  Pi1/LConn1 -- a_in/RConn1
  Pi2/LConn1 -- b_in/RConn1
  Pi3/LConn1 -- c_in/RConn1
  Pi3/RConn1 -- c_out/RConn1
  Pi4/RConn1 -- d_out/RConn1
  Pi4/LConn1 -- d_in/RConn1

== system typhoonPatterns/PMSM ==
  mech : Inport
  PMSM1 : powerlib/Machines/Permanent Magnet Synchronous Machine  NbPhases=3  FluxDistribution=Sinusoidal  RotorType=Salient-pole  MechanicalLoad=Speed w  PresetModel=No  ShowDetailedParameters=on  MeasurementBus=on  Resistance=Rs  Inductance=8.5e-3  dqInductances=[Ld, Lq]  La=Lms  MachineConstant=Flux linkage established by magnets (V.s)  Flux=psi_pm  VoltageCst=86.6271  TorqueCst=0.7164  Flat=120  Mechanical=[Jm fc pms 0]  PolePairs=pms  InitialConditions=[0,0, 0,0]  InitialConditions5ph=[0 0 0 0 0 0]  TsPowergui=0  TsBlock=-1  RefAngle=90 degrees behind phase A axis (modified Park)
      settings: SourceProductName=Simscape Power Systems
  A : PMIOPort  Port=1  Side=Left
  B : PMIOPort  Port=2  Side=Left
  C : PMIOPort  Port=3  Side=Left
  meas : Outport
  wires:
  mech/1 -> PMSM1/1
  PMSM1/1 -> meas/1
  connections:
  A/RConn1 -- PMSM1/LConn1
  B/RConn1 -- PMSM1/LConn2
  C/RConn1 -- PMSM1/LConn3

== system typhoonPatterns/RL Coupled 2PH ==
  RL1 : powerlib/Elements/Series RLC Branch  LConnTagsString=__new0  RConnTagsString=__new0  BranchType=RL  Resistance=R  Inductance=L  SetiL0=off  InitialCurrent=0  Capacitance=1e-6  Setx0=off  InitialVoltage=0  Measurements=None
  RL2 : powerlib/Elements/Series RLC Branch  LConnTagsString=__new0  RConnTagsString=__new0  BranchType=RL  Resistance=R  Inductance=L  SetiL0=off  InitialCurrent=0  Capacitance=1e-6  Setx0=off  InitialVoltage=0  Measurements=None
  a_in : PMIOPort  Port=1  Side=Left
  a_out : PMIOPort  Port=2  Side=Right
  b_in : PMIOPort  Port=3  Side=Left
  b_out : PMIOPort  Port=4  Side=Right
  connections:
  b_in/RConn1 -- RL2/LConn1
  a_in/RConn1 -- RL1/LConn1
  a_out/RConn1 -- RL1/RConn1
  b_out/RConn1 -- RL2/RConn1

== system typhoonPatterns/RL Coupled 3PH ==
  RL1 : powerlib/Elements/Series RLC Branch  LConnTagsString=__new0  RConnTagsString=__new0  BranchType=RL  Resistance=R  Inductance=L  SetiL0=off  InitialCurrent=0  Capacitance=1e-6  Setx0=off  InitialVoltage=0  Measurements=None
  RL2 : powerlib/Elements/Series RLC Branch  LConnTagsString=__new0  RConnTagsString=__new0  BranchType=RL  Resistance=R  Inductance=L  SetiL0=off  InitialCurrent=0  Capacitance=1e-6  Setx0=off  InitialVoltage=0  Measurements=None
  RL3 : powerlib/Elements/Series RLC Branch  LConnTagsString=__new0  RConnTagsString=__new0  BranchType=RL  Resistance=R  Inductance=L  SetiL0=off  InitialCurrent=0  Capacitance=1e-6  Setx0=off  InitialVoltage=0  Measurements=None
  a_in : PMIOPort  Port=1  Side=Left
  a_out : PMIOPort  Port=2  Side=Right
  b_in : PMIOPort  Port=3  Side=Left
  b_out : PMIOPort  Port=4  Side=Right
  c_in : PMIOPort  Port=5  Side=Left
  c_out : PMIOPort  Port=6  Side=Right
  connections:
  b_out/RConn1 -- RL2/RConn1
  a_out/RConn1 -- RL1/RConn1
  a_in/RConn1 -- RL1/LConn1
  b_in/RConn1 -- RL2/LConn1
  c_in/RConn1 -- RL3/LConn1
  c_out/RConn1 -- RL3/RConn1

== system typhoonPatterns/RL Coupled 4PH ==
  RL{1..4} (4 alike) : powerlib/Elements/Series RLC Branch  LConnTagsString=__new0  RConnTagsString=__new0  BranchType=RL  Resistance=R  Inductance=L  SetiL0=off  InitialCurrent=0  Capacitance=1e-6  Setx0=off  InitialVoltage=0  Measurements=None
  a_in : PMIOPort  Port=1  Side=Left
  a_out : PMIOPort  Port=2  Side=Right
  b_in : PMIOPort  Port=3  Side=Left
  b_out : PMIOPort  Port=4  Side=Right
  c_in : PMIOPort  Port=5  Side=Left
  c_out : PMIOPort  Port=6  Side=Right
  d_in : PMIOPort  Port=7  Side=Left
  d_out : PMIOPort  Port=8  Side=Right
  connections:
  d_in/RConn1 -- RL4/LConn1
  d_out/RConn1 -- RL4/RConn1
  c_out/RConn1 -- RL3/RConn1
  c_in/RConn1 -- RL3/LConn1
  b_in/RConn1 -- RL2/LConn1
  a_in/RConn1 -- RL1/LConn1
  a_out/RConn1 -- RL1/RConn1
  b_out/RConn1 -- RL2/RConn1

== system typhoonPatterns/RL Section 1PH ==
  RL1 : powerlib/Elements/Series RLC Branch  LConnTagsString=__new0  RConnTagsString=__new0  BranchType=RL  Resistance=R  Inductance=L  SetiL0=off  InitialCurrent=0  Capacitance=1e-6  Setx0=off  InitialVoltage=0  Measurements=None
  a_in : PMIOPort  Port=1  Side=Left
  a_out : PMIOPort  Port=2  Side=Right
  connections:
  a_in/RConn1 -- RL1/LConn1
  a_out/RConn1 -- RL1/RConn1

== system typhoonPatterns/RL Section 2PH ==
  RL1 : powerlib/Elements/Series RLC Branch  LConnTagsString=__new0  RConnTagsString=__new0  BranchType=RL  Resistance=R  Inductance=L  SetiL0=off  InitialCurrent=0  Capacitance=1e-6  Setx0=off  InitialVoltage=0  Measurements=None
  RL2 : powerlib/Elements/Series RLC Branch  LConnTagsString=__new0  RConnTagsString=__new0  BranchType=RL  Resistance=R  Inductance=L  SetiL0=off  InitialCurrent=0  Capacitance=1e-6  Setx0=off  InitialVoltage=0  Measurements=None
  a_in : PMIOPort  Port=1  Side=Left
  a_out : PMIOPort  Port=2  Side=Right
  b_in : PMIOPort  Port=3  Side=Left
  b_out : PMIOPort  Port=4  Side=Right
  connections:
  b_out/RConn1 -- RL2/RConn1
  a_out/RConn1 -- RL1/RConn1
  a_in/RConn1 -- RL1/LConn1
  b_in/RConn1 -- RL2/LConn1

== system typhoonPatterns/RL Section 3PH ==
  RL1 : powerlib/Elements/Series RLC Branch  LConnTagsString=__new0  RConnTagsString=__new0  BranchType=RL  Resistance=R  Inductance=L  SetiL0=off  InitialCurrent=0  Capacitance=1e-6  Setx0=off  InitialVoltage=0  Measurements=None
  RL2 : powerlib/Elements/Series RLC Branch  LConnTagsString=__new0  RConnTagsString=__new0  BranchType=RL  Resistance=R  Inductance=L  SetiL0=off  InitialCurrent=0  Capacitance=1e-6  Setx0=off  InitialVoltage=0  Measurements=None
  RL3 : powerlib/Elements/Series RLC Branch  LConnTagsString=__new0  RConnTagsString=__new0  BranchType=RL  Resistance=R  Inductance=L  SetiL0=off  InitialCurrent=0  Capacitance=1e-6  Setx0=off  InitialVoltage=0  Measurements=None
  a_in : PMIOPort  Port=1  Side=Left
  a_out : PMIOPort  Port=2  Side=Right
  b_in : PMIOPort  Port=3  Side=Left
  b_out : PMIOPort  Port=4  Side=Right
  c_in : PMIOPort  Port=5  Side=Left
  c_out : PMIOPort  Port=6  Side=Right
  connections:
  c_out/RConn1 -- RL3/RConn1
  c_in/RConn1 -- RL3/LConn1
  b_in/RConn1 -- RL2/LConn1
  a_in/RConn1 -- RL1/LConn1
  a_out/RConn1 -- RL1/RConn1
  b_out/RConn1 -- RL2/RConn1

== system typhoonPatterns/RL Section 4PH ==
  RL{1..4} (4 alike) : powerlib/Elements/Series RLC Branch  LConnTagsString=__new0  RConnTagsString=__new0  BranchType=RL  Resistance=R  Inductance=L  SetiL0=off  InitialCurrent=0  Capacitance=1e-6  Setx0=off  InitialVoltage=0  Measurements=None
  a_in : PMIOPort  Port=1  Side=Left
  a_out : PMIOPort  Port=2  Side=Right
  b_in : PMIOPort  Port=3  Side=Left
  b_out : PMIOPort  Port=4  Side=Right
  c_in : PMIOPort  Port=5  Side=Left
  c_out : PMIOPort  Port=6  Side=Right
  d_in : PMIOPort  Port=7  Side=Left
  d_out : PMIOPort  Port=8  Side=Right
  connections:
  b_out/RConn1 -- RL2/RConn1
  a_out/RConn1 -- RL1/RConn1
  a_in/RConn1 -- RL1/LConn1
  b_in/RConn1 -- RL2/LConn1
  c_in/RConn1 -- RL3/LConn1
  c_out/RConn1 -- RL3/RConn1
  d_out/RConn1 -- RL4/RConn1
  d_in/RConn1 -- RL4/LConn1

== system typhoonPatterns/RL Section 5PH ==
  RL{1..5} (5 alike) : powerlib/Elements/Series RLC Branch  LConnTagsString=__new0  RConnTagsString=__new0  BranchType=RL  Resistance=R  Inductance=L  SetiL0=off  InitialCurrent=0  Capacitance=1e-6  Setx0=off  InitialVoltage=0  Measurements=None
  a_in : PMIOPort  Port=1  Side=Left
  a_out : PMIOPort  Port=2  Side=Right
  b_in : PMIOPort  Port=3  Side=Left
  b_out : PMIOPort  Port=4  Side=Right
  c_in : PMIOPort  Port=5  Side=Left
  c_out : PMIOPort  Port=6  Side=Right
  d_in : PMIOPort  Port=7  Side=Left
  d_out : PMIOPort  Port=8  Side=Right
  e_in : PMIOPort  Port=9  Side=Left
  e_out : PMIOPort  Port=10  Side=Right
  connections:
  d_in/RConn1 -- RL4/LConn1
  d_out/RConn1 -- RL4/RConn1
  c_out/RConn1 -- RL3/RConn1
  c_in/RConn1 -- RL3/LConn1
  b_in/RConn1 -- RL2/LConn1
  a_in/RConn1 -- RL1/LConn1
  a_out/RConn1 -- RL1/RConn1
  b_out/RConn1 -- RL2/RConn1
  e_out/RConn1 -- RL5/RConn1
  e_in/RConn1 -- RL5/LConn1

== system typhoonPatterns/SP 2W Transformer ==
  T1 : powerlib/Elements/Multi-Winding Transformer  LeftWindings=1  RightWindings=1  TappedWindings=no taps  NumberOfTaps=2  SetSaturation=off  Hysteresis=off  DataFile='hysteresis.mat'  Measurements=None  UNITS=SI  NominalPower=[1, 1]  NominalVoltages=[1,1]  WindingResistances=[1 1]  WindingInductances=[1,1]  Rm=1  Lm=1  Saturation=[0 0;0.0033941 0.27009;1.4142 0.34212]  MoreParameters=off  BreakLoop=off  DataType=on  InitialFlux=0  TransfoNumber=1
      settings: AttributesFormatString=%<MaskType>  SourceProductName=Simscape Power Systems  SourceProductBaseCode=PS
  prm_1 : PMIOPort  Port=1  Side=Left
  prm_2 : PMIOPort  Port=2  Side=Left
  sec_1 : PMIOPort  Port=3  Side=Right
  sec_2 : PMIOPort  Port=4  Side=Right
  connections:
  sec_1/RConn1 -- T1/RConn1
  sec_2/RConn1 -- T1/RConn2
  prm_1/RConn1 -- T1/LConn1
  prm_2/RConn1 -- T1/LConn2

== system typhoonPatterns/SP 3W Transformer ==
  T1 : powerlib/Elements/Multi-Winding Transformer  LeftWindings=1  RightWindings=2  TappedWindings=no taps  NumberOfTaps=2  SetSaturation=off  Hysteresis=off  DataFile='hysteresis.mat'  Measurements=None  UNITS=SI  NominalPower=[1,1]  NominalVoltages=[1,1,1]  WindingResistances=[1 1 1]  WindingInductances=[1,1,1,1]  Rm=1  Lm=1  Saturation=[0 0;0.0033941 0.27009;1.4142 0.34212]  MoreParameters=off  BreakLoop=off  DataType=on  InitialFlux=0  TransfoNumber=1
      settings: AttributesFormatString=%<MaskType>  SourceProductName=Simscape Power Systems  SourceProductBaseCode=PS
  prm_1 : PMIOPort  Port=1  Side=Left
  prm_2 : PMIOPort  Port=2  Side=Left
  sec_1 : PMIOPort  Port=3  Side=Right
  sec_2 : PMIOPort  Port=4  Side=Right
  sec_3 : PMIOPort  Port=5  Side=Right
  sec_4 : PMIOPort  Port=6  Side=Right
  connections:
  sec_2/RConn1 -- T1/RConn2
  T1/LConn2 -- prm_2/RConn1
  T1/RConn1 -- sec_1/RConn1
  T1/LConn1 -- prm_1/RConn1
  T1/RConn3 -- sec_3/RConn1
  T1/RConn4 -- sec_4/RConn1

== system typhoonPatterns/SP 4W Transformer ==
  T1 : powerlib/Elements/Multi-Winding Transformer  LeftWindings=1  RightWindings=3  TappedWindings=no taps  NumberOfTaps=2  SetSaturation=off  Hysteresis=off  DataFile='hysteresis.mat'  Measurements=None  UNITS=SI  NominalPower=[1, 1]  NominalVoltages=[1,1,1,1]  WindingResistances=[1 1 1 1]  WindingInductances=[1 1 1 1]  Rm=1  Lm=1  Saturation=[0 0;0.0048 0.060792;2 0.077004]  MoreParameters=off  BreakLoop=off  DataType=on  InitialFlux=0  TransfoNumber=1
      settings: AttributesFormatString=%<MaskType>  SourceProductName=Simscape Power Systems  SourceProductBaseCode=PS
  prm_1 : PMIOPort  Port=1  Side=Left
  prm_2 : PMIOPort  Port=2  Side=Left
  sec_1 : PMIOPort  Port=3  Side=Right
  sec_2 : PMIOPort  Port=4  Side=Right
  sec_3 : PMIOPort  Port=5  Side=Right
  sec_4 : PMIOPort  Port=6  Side=Right
  sec_5 : PMIOPort  Port=7  Side=Right
  sec_6 : PMIOPort  Port=8  Side=Right
  connections:
  T1/RConn4 -- sec_4/RConn1
  T1/RConn3 -- sec_3/RConn1
  T1/LConn1 -- prm_1/RConn1
  T1/RConn1 -- sec_1/RConn1
  T1/LConn2 -- prm_2/RConn1
  sec_2/RConn1 -- T1/RConn2
  T1/RConn5 -- sec_5/RConn1
  T1/RConn6 -- sec_6/RConn1

== system typhoonPatterns/SP CC ==
  a_in : PMIOPort  Port=1  Side=Left
  b_in : PMIOPort  Port=2  Side=Left
  a_out : PMIOPort  Port=3  Side=Right
  b_out : PMIOPort  Port=4  Side=Right
  connections:
  a_in/RConn1 -- a_out/RConn1
  b_in/RConn1 -- b_out/RConn1

== system typhoonPatterns/SP Induction Machine ==
  mech : Inport
  SP Asynchronous Machine1 : powerlib/Machines/Single Phase Asynchronous Machine  MechanicalLoad=Torque Tm  UNITS=SI  MachineType=Split Phase  MeasurementBus=off  NominalParameters="[0  0  f_sp_ind]"  MainWindingStator="[rsm_sp_ind  llsm_sp_ind]"  MainWindingRotor="[rrm_sp_ind  llrm_sp_ind]"  MutualInductance=lmm_sp_ind  AuxiliaryWinding="[rsa_sp_ind  llsa_sp_ind]"  Mechanical="[Jm  fc pms nanm_sp_ind]"  CapacitorStart="[rst_sp_ind  cst_sp_ind]"  CapacitorRun=[rrun_sp_ind crun_sp_ind]  DisconnectionSpeed=w_disc  InitialSpeed=0  DataType=SI  TsPowergui=0  TsBlock=-1
      settings: SourceProductName=Simscape Power Systems  SourceProductBaseCode=PS
  A : PMIOPort  Port=1  Side=Left
  B : PMIOPort  Port=2  Side=Left
  meas : Outport
  wires:
  mech/1 -> SP Asynchronous Machine1/1
  SP Asynchronous Machine1/1 -> meas/1
  connections:
  SP Asynchronous Machine1/LConn1 -- A/RConn1
  SP Asynchronous Machine1/LConn2 -- B/RConn1

== system typhoonPatterns/SPDT Contactor ==
  control : Inport
  Sa_1 : powerlib/Power Electronics/Ideal Switch  Ron=r_on  Lon=0  IC=s0  Rs=r_s  Cs=c_s  Measurements=on
  Sa_2 : powerlib/Power Electronics/Ideal Switch  Ron=r_on  Lon=0  IC=s0  Rs=r_s  Cs=c_s  Measurements=on
  inv1 : Logic  Commented=through  Operator=NOT  AllPortsSameDT=off  OutDataTypeStr=boolean
  inv2 : Logic  Operator=NOT  AllPortsSameDT=off  OutDataTypeStr=boolean
  A : PMIOPort  Port=1  Side=Left
  B : PMIOPort  Port=2  Side=Left
  C : PMIOPort  Port=3  Side=Right
  wires:
  inv1/1 -> inv2/1, [S_1]
  control/1 -> inv1/1
  inv2/1 -> [S_2]
  [S_1] -> Sa_1/1
  [S_2] -> Sa_2/1
  connections:
  A/RConn1 -- Sa_1/LConn1
  B/RConn1 -- Sa_2/LConn1
  C/RConn1 -- Sa_1/RConn1 -- Sa_2/RConn1

== system typhoonPatterns/SPST Contactor ==
  control : Inport
  Sa : powerlib/Power Electronics/Ideal Switch  Ron=r_on  Lon=0  IC=s0  Rs=r_s  Cs=c_s  Measurements=on
  inv1 : Logic  Commented=through  Operator=NOT  AllPortsSameDT=off  OutDataTypeStr=boolean
  A : PMIOPort  Port=1  Side=Left
  B : PMIOPort  Port=2  Side=Right
  wires:
  control/1 -> inv1/1
  inv1/1 -> Sa/1
  connections:
  B/RConn1 -- Sa/RConn1
  A/RConn1 -- Sa/LConn1
